simulink model "dp_controller"  (R2020a)
settings: Solver=FixedStepAuto  StartTime=0.0  StopTime=10.0  FixedStep=0.01  RelTol=1e-3
PreLoadFcn:
  | load("interfaces.mat");
undefined symbols (not defined in the file or in its folder): surge, sway, yaw
libraries: simulink x3
settings Model: Creator=thomas.evang  LastModifiedBy=thomas.evang
settings SFSimCC: CustomCodeUndefinedFunction=UseInterfaceOnly
settings RTWCC: Description=Generic Real-Time Target  RetainRTWFile=on

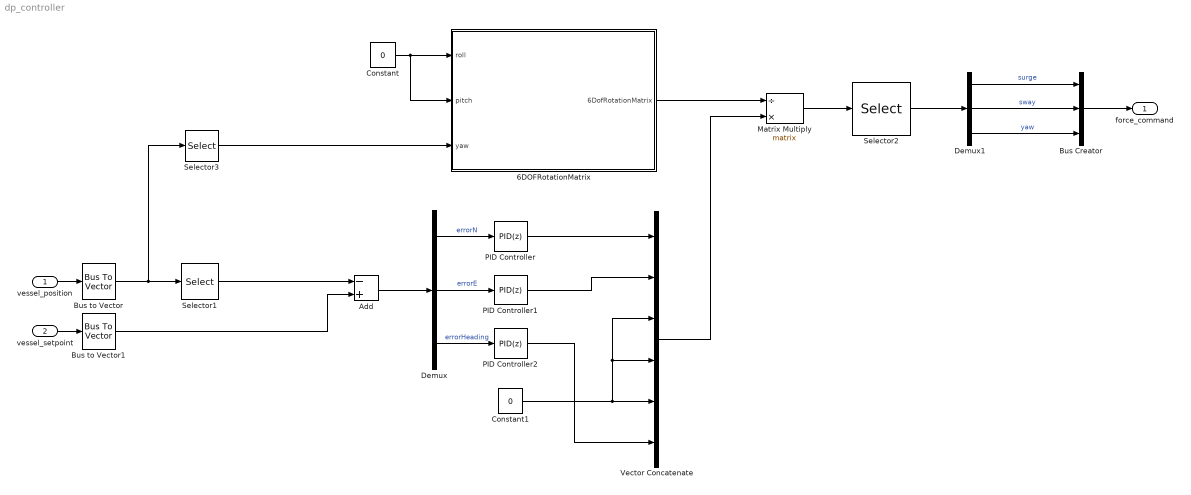
== system dp_controller ==
  vessel_position : Inport  OutDataTypeStr=Bus: position_6dof
  vessel_setpoint : Inport  Port=2  OutDataTypeStr=Bus: position_3dof
  6DOFRotationMatrix : Subsystem
  Add : Sum  Inputs=-+
  Bus Creator : BusCreator  Inputs=surge,sway,yaw  OutDataTypeStr=Bus: force_3dof
  Bus to Vector : BusToVector
  Bus to Vector1 : BusToVector
  Constant : Constant  Value=0
  Constant1 : Constant  Value=0
  Demux : Demux  Outputs=3
  Demux1 : Demux  Outputs=3
  Matrix Multiply : Product  Inputs=/*  Multiplication=Matrix(*)
  PID Controller : simulink/Continuous/PID Controller  Controller=PID  Form=Parallel  TimeDomain=Discrete-time  UseExternalTs=off  SampleTime=1e-1  IntegratorMethod=Forward Euler  FilterMethod=Forward Euler  ControllerParametersSource=internal  P=50000  I=100  D=5000000  UseFilter=off  N=0  TunerSelectOption=Transfer Function Based (PID Tuner App)  InitialConditionSource=internal  InitialConditionForIntegrator=0  InitialConditionForFilter=0  DifferentiatorICPrevScaledInput=0  ExternalReset=none  TrackingMode=off  Kt=1  LimitOutput=off  UpperSaturationLimit=inf  LowerSaturationLimit=-inf  LinearizeAsGain=on  AntiWindupMode=none  Kb=1  POutMin=[]  POutMax=[]  IOutMin=[]  IOutMax=[]  DOutMin=[]  DOutMax=[]  NOutMin=[]  NOutMax=[]  SumOutMin=[]  SumOutMax=[]  SaturationOutMin=[]  SaturationOutMax=[]  PParamMin=[]  PParamMax=[]  IParamMin=[]  IParamMax=[]  DParamMin=[]  DParamMax=[]  NParamMin=[]  NParamMax=[]  KbParamMin=[]  KbParamMax=[]  KtParamMin=[]  KtParamMax=[]  KbOutMin=[]  KbOutMax=[]  KtOutMin=[]  KtOutMax=[]  IntegratorOutMin=[]  IntegratorOutMax=[]  FilterOutMin=[]  FilterOutMax=[]  SumI1OutMin=[]  SumI1OutMax=[]  SumI2OutMin=[]  SumI2OutMax=[]  SumI3OutMin=[]  SumI3OutMax=[]  SumI4OutMin=[]  SumI4OutMax=[]  SumDOutMin=[]  SumDOutMax=[]  DifferentiatorOutMin=[]  DifferentiatorOutMax=[]  FilterDiffOutCoefMin=[]  FilterDiffOutCoefMax=[]  ReciprocalOutMin=[]  ReciprocalOutMax=[]  SumDenOutMin=[]  SumDenOutMax=[]  SumNumOutMin=[]  SumNumOutMax=[]  DivideOutMin=[]  DivideOutMax=[]  UdiffTsProdOutMin=[]  UdiffTsProdOutMax=[]  NTsProdOutMin=[]  NTsProdOutMax=[]  UintegralTsProdOutMin=[]  UintegralTsProdOutMax=[]  UngainTsProdOutMin=[]  UngainTsProdOutMax=[]  IntegratorContinuousStateAttributes=''  IntegratorStateMustResolveToSignalObject=off  IntegratorRTWStateStorageClass=Auto  FilterContinuousStateAttributes=''  FilterStateMustResolveToSignalObject=off  FilterRTWStateStorageClass=Auto  ParallelPVariant=InternalParameters  IdealPVariant=Disabled  IVariant=InternalParameters  DVariant=InternalParameters  IntegratorVariant=Discrete  SatVariant=Disabled  AWVariant=Passthrough  PCopyVariant=Disabled  TRVariant=Disabled  FdbkBlocksVariant=Forward  IdealPFdbkVariant=Disabled  SatFdbkVariant=Disabled  DerivativeFilterVariant=Differentiator  NVariant=Passthrough  NCopyVariant=Disabled_SignalSpec  FilterICVariant=InternalICsDifferentiator  IntegratorICVariant=InternalICs  ExternalResetVariant=Disabled  TRSumVariant=Passthrough  SumFdbkVariant=Disabled  SumVariant=Sum_PID  TsampFilterVariant=InternalTs  TsampNgainVariant=Passthrough  TsampIntegralVariant=Passthrough
  PID Controller1 : simulink/Continuous/PID Controller  Controller=PID  Form=Parallel  TimeDomain=Discrete-time  UseExternalTs=off  SampleTime=1e-1  IntegratorMethod=Forward Euler  FilterMethod=Forward Euler  ControllerParametersSource=internal  P=50000  I=100  D=5000000  UseFilter=off  N=0  TunerSelectOption=Transfer Function Based (PID Tuner App)  InitialConditionSource=internal  InitialConditionForIntegrator=0  InitialConditionForFilter=0  DifferentiatorICPrevScaledInput=0  ExternalReset=none  TrackingMode=off  Kt=1  LimitOutput=off  UpperSaturationLimit=inf  LowerSaturationLimit=-inf  LinearizeAsGain=on  AntiWindupMode=none  Kb=1  POutMin=[]  POutMax=[]  IOutMin=[]  IOutMax=[]  DOutMin=[]  DOutMax=[]  NOutMin=[]  NOutMax=[]  SumOutMin=[]  SumOutMax=[]  SaturationOutMin=[]  SaturationOutMax=[]  PParamMin=[]  PParamMax=[]  IParamMin=[]  IParamMax=[]  DParamMin=[]  DParamMax=[]  NParamMin=[]  NParamMax=[]  KbParamMin=[]  KbParamMax=[]  KtParamMin=[]  KtParamMax=[]  KbOutMin=[]  KbOutMax=[]  KtOutMin=[]  KtOutMax=[]  IntegratorOutMin=[]  IntegratorOutMax=[]  FilterOutMin=[]  FilterOutMax=[]  SumI1OutMin=[]  SumI1OutMax=[]  SumI2OutMin=[]  SumI2OutMax=[]  SumI3OutMin=[]  SumI3OutMax=[]  SumI4OutMin=[]  SumI4OutMax=[]  SumDOutMin=[]  SumDOutMax=[]  DifferentiatorOutMin=[]  DifferentiatorOutMax=[]  FilterDiffOutCoefMin=[]  FilterDiffOutCoefMax=[]  ReciprocalOutMin=[]  ReciprocalOutMax=[]  SumDenOutMin=[]  SumDenOutMax=[]  SumNumOutMin=[]  SumNumOutMax=[]  DivideOutMin=[]  DivideOutMax=[]  UdiffTsProdOutMin=[]  UdiffTsProdOutMax=[]  NTsProdOutMin=[]  NTsProdOutMax=[]  UintegralTsProdOutMin=[]  UintegralTsProdOutMax=[]  UngainTsProdOutMin=[]  UngainTsProdOutMax=[]  IntegratorContinuousStateAttributes=''  IntegratorStateMustResolveToSignalObject=off  IntegratorRTWStateStorageClass=Auto  FilterContinuousStateAttributes=''  FilterStateMustResolveToSignalObject=off  FilterRTWStateStorageClass=Auto  ParallelPVariant=InternalParameters  IdealPVariant=Disabled  IVariant=InternalParameters  DVariant=InternalParameters  IntegratorVariant=Discrete  SatVariant=Disabled  AWVariant=Passthrough  PCopyVariant=Disabled  TRVariant=Disabled  FdbkBlocksVariant=Forward  IdealPFdbkVariant=Disabled  SatFdbkVariant=Disabled  DerivativeFilterVariant=Differentiator  NVariant=Passthrough  NCopyVariant=Disabled_SignalSpec  FilterICVariant=InternalICsDifferentiator  IntegratorICVariant=InternalICs  ExternalResetVariant=Disabled  TRSumVariant=Passthrough  SumFdbkVariant=Disabled  SumVariant=Sum_PID  TsampFilterVariant=InternalTs  TsampNgainVariant=Passthrough  TsampIntegralVariant=Passthrough
  PID Controller2 : simulink/Continuous/PID Controller  Controller=PID  Form=Parallel  TimeDomain=Discrete-time  UseExternalTs=off  SampleTime=1e-1  IntegratorMethod=Forward Euler  FilterMethod=Forward Euler  ControllerParametersSource=internal  P=987355.105195486  I=621.647398453693  D=34853426.651765  UseFilter=off  N=100  TunerSelectOption=Transfer Function Based (PID Tuner App)  InitialConditionSource=internal  InitialConditionForIntegrator=0  InitialConditionForFilter=0  DifferentiatorICPrevScaledInput=0  ExternalReset=none  TrackingMode=off  Kt=1  LimitOutput=off  UpperSaturationLimit=inf  LowerSaturationLimit=-inf  LinearizeAsGain=on  AntiWindupMode=none  Kb=1  POutMin=[]  POutMax=[]  IOutMin=[]  IOutMax=[]  DOutMin=[]  DOutMax=[]  NOutMin=[]  NOutMax=[]  SumOutMin=[]  SumOutMax=[]  SaturationOutMin=[]  SaturationOutMax=[]  PParamMin=[]  PParamMax=[]  IParamMin=[]  IParamMax=[]  DParamMin=[]  DParamMax=[]  NParamMin=[]  NParamMax=[]  KbParamMin=[]  KbParamMax=[]  KtParamMin=[]  KtParamMax=[]  KbOutMin=[]  KbOutMax=[]  KtOutMin=[]  KtOutMax=[]  IntegratorOutMin=[]  IntegratorOutMax=[]  FilterOutMin=[]  FilterOutMax=[]  SumI1OutMin=[]  SumI1OutMax=[]  SumI2OutMin=[]  SumI2OutMax=[]  SumI3OutMin=[]  SumI3OutMax=[]  SumI4OutMin=[]  SumI4OutMax=[]  SumDOutMin=[]  SumDOutMax=[]  DifferentiatorOutMin=[]  DifferentiatorOutMax=[]  FilterDiffOutCoefMin=[]  FilterDiffOutCoefMax=[]  ReciprocalOutMin=[]  ReciprocalOutMax=[]  SumDenOutMin=[]  SumDenOutMax=[]  SumNumOutMin=[]  SumNumOutMax=[]  DivideOutMin=[]  DivideOutMax=[]  UdiffTsProdOutMin=[]  UdiffTsProdOutMax=[]  NTsProdOutMin=[]  NTsProdOutMax=[]  UintegralTsProdOutMin=[]  UintegralTsProdOutMax=[]  UngainTsProdOutMin=[]  UngainTsProdOutMax=[]  IntegratorContinuousStateAttributes=''  IntegratorStateMustResolveToSignalObject=off  IntegratorRTWStateStorageClass=Auto  FilterContinuousStateAttributes=''  FilterStateMustResolveToSignalObject=off  FilterRTWStateStorageClass=Auto  ParallelPVariant=InternalParameters  IdealPVariant=Disabled  IVariant=InternalParameters  DVariant=InternalParameters  IntegratorVariant=Discrete  SatVariant=Disabled  AWVariant=Passthrough  PCopyVariant=Disabled  TRVariant=Disabled  FdbkBlocksVariant=Forward  IdealPFdbkVariant=Disabled  SatFdbkVariant=Disabled  DerivativeFilterVariant=Differentiator  NVariant=Passthrough  NCopyVariant=Disabled_SignalSpec  FilterICVariant=InternalICsDifferentiator  IntegratorICVariant=InternalICs  ExternalResetVariant=Disabled  TRSumVariant=Passthrough  SumFdbkVariant=Disabled  SumVariant=Sum_PID  TsampFilterVariant=InternalTs  TsampNgainVariant=Passthrough  TsampIntegralVariant=Passthrough
  Selector1 : Selector  InputPortWidth=6  IndexOptions=Index vector (dialog)  Indices=[1 2 6]  OutputSizes=1
  Selector2 : Selector  InputPortWidth=6  IndexOptions=Index vector (dialog)  Indices=[1 2 6]  OutputSizes=1
  Selector3 : Selector  InputPortWidth=6  IndexOptions=Index vector (dialog)  Indices=6  OutputSizes=1
  Vector Concatenate : Concatenate  NumInputs=6
  force_command : Outport  OutDataTypeStr=Bus: force_3dof  VectorParamsAs1DForOutWhenUnconnected=off
  wires:
  Selector1/1 -> Add/1
  PID Controller2/1 -> Vector Concatenate/6
  Matrix Multiply/1 -> Selector2/1
  Selector3/1 -> 6DOFRotationMatrix/3(yaw)
  Demux/1 -> PID Controller/1  "errorN"
  Demux/3 -> PID Controller2/1  "errorHeading"
  PID Controller/1 -> Vector Concatenate/1
  Add/1 -> Demux/1
  Constant/1 -> 6DOFRotationMatrix/1(roll), 6DOFRotationMatrix/2(pitch)
  vessel_setpoint/1 -> Bus to Vector1/1
  Constant1/1 -> Vector Concatenate/5, Vector Concatenate/3, Vector Concatenate/4
  PID Controller1/1 -> Vector Concatenate/2
  vessel_position/1 -> Bus to Vector/1
  Demux/2 -> PID Controller1/1  "errorE"
  Vector Concatenate/1 -> Matrix Multiply/2
  6DOFRotationMatrix/1(6DofRotationMatrix) -> Matrix Multiply/1
  Selector2/1 -> Demux1/1
  Bus Creator/1 -> force_command/1
  Demux1/1 -> Bus Creator/1  "surge"
  Demux1/2 -> Bus Creator/2  "sway"
  Demux1/3 -> Bus Creator/3  "yaw"
  Bus to Vector/1 -> Selector3/1, Selector1/1
  Bus to Vector1/1 -> Add/2

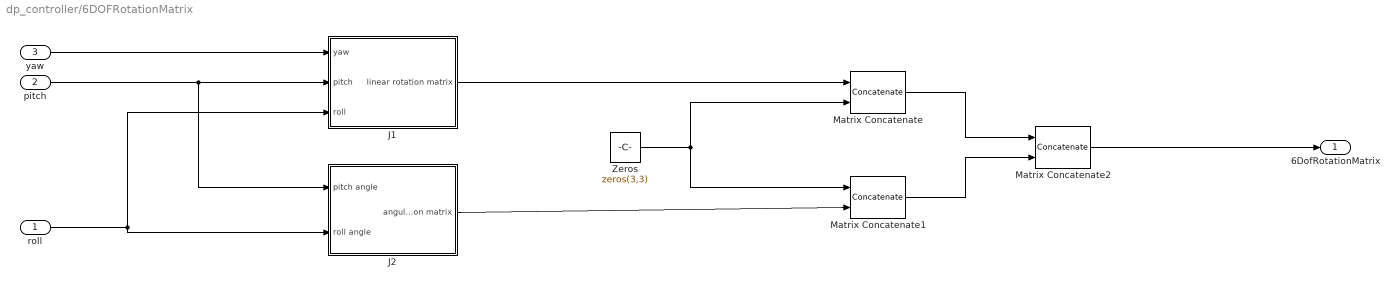
== system dp_controller/6DOFRotationMatrix ==
  roll : Inport
  pitch : Inport  Port=2
  yaw : Inport  Port=3
  J1 : Subsystem
  J2 : Subsystem
  Matrix Concatenate : Concatenate  Mode=Multidimensional array
  Matrix Concatenate1 : Concatenate  Mode=Multidimensional array
  Matrix Concatenate2 : Concatenate  Mode=Multidimensional array  ConcatenateDimension=2
  Zeros : Constant  Value=zeros(3,3)
  6DofRotationMatrix : Outport  VectorParamsAs1DForOutWhenUnconnected=off
  wires:
  J1/1(linear rotation matrix) -> Matrix Concatenate/1
  yaw/1 -> J1/1(yaw)
  J2/1(angular rotation matrix) -> Matrix Concatenate1/2
  Matrix Concatenate2/1 -> 6DofRotationMatrix/1
  Matrix Concatenate/1 -> Matrix Concatenate2/1
  Matrix Concatenate1/1 -> Matrix Concatenate2/2
  Zeros/1 -> Matrix Concatenate1/1, Matrix Concatenate/2
  roll/1 -> J2/2(roll angle), J1/3(roll)
  pitch/1 -> J1/2(pitch), J2/1(pitch angle)

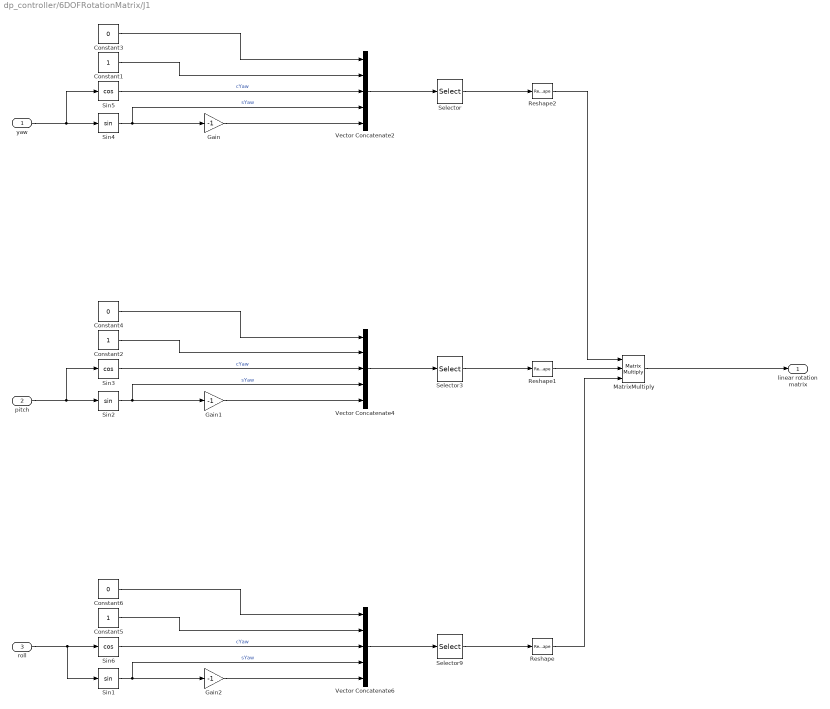
== system dp_controller/6DOFRotationMatrix/J1 ==
  yaw : Inport
  pitch : Inport  Port=2
  roll : Inport  Port=3
  Constant1 : Constant
  Constant2 : Constant
  Constant3 : Constant  Value=0
  Constant4 : Constant  Value=0
  Constant5 : Constant
  Constant6 : Constant  Value=0
  Gain : Gain  Gain=-1
  Gain1 : Gain  Gain=-1
  Gain2 : Gain  Gain=-1
  MatrixMultiply : Product  Inputs=3  Multiplication=Matrix(*)
  Reshape : Reshape  OutputDimensionality=Customize  OutputDimensions=[3,3]
  Reshape1 : Reshape  OutputDimensionality=Customize  OutputDimensions=[3,3]
  Reshape2 : Reshape  OutputDimensionality=Customize  OutputDimensions=[3,3]
  Selector : Selector  InputPortWidth=5  IndexOptions=Index vector (dialog)  Indices=[3 4 1 5 3 1 1 1 2]  OutputSizes=1
  Selector3 : Selector  InputPortWidth=5  IndexOptions=Index vector (dialog)  Indices=[3 1 5 1 2 1 4 1 3]  OutputSizes=1
  Selector9 : Selector  InputPortWidth=5  IndexOptions=Index vector (dialog)  Indices=[2 1 1 1 3 4 1 5 3]  OutputSizes=1
  Sin1 : Trigonometry
  Sin2 : Trigonometry
  Sin3 : Trigonometry  Operator=cos
  Sin4 : Trigonometry
  Sin5 : Trigonometry  Operator=cos
  Sin6 : Trigonometry  Operator=cos
  Vector Concatenate2 : Concatenate  NumInputs=5
  Vector Concatenate4 : Concatenate  NumInputs=5
  Vector Concatenate6 : Concatenate  NumInputs=5
  linear rotation matrix : Outport  VectorParamsAs1DForOutWhenUnconnected=off
  wires:
  Sin5/1 -> Vector Concatenate2/3  "cYaw"
  Constant3/1 -> Vector Concatenate2/1
  Constant2/1 -> Vector Concatenate4/2
  Constant4/1 -> Vector Concatenate4/1
  Gain1/1 -> Vector Concatenate4/5
  roll/1 -> Sin6/1, Sin1/1
  Constant1/1 -> Vector Concatenate2/2
  Vector Concatenate4/1 -> Selector3/1
  Vector Concatenate2/1 -> Selector/1
  Reshape2/1 -> MatrixMultiply/1
  Gain/1 -> Vector Concatenate2/5
  Selector9/1 -> Reshape/1
  Vector Concatenate6/1 -> Selector9/1
  Gain2/1 -> Vector Concatenate6/5
  Reshape1/1 -> MatrixMultiply/2
  Selector3/1 -> Reshape1/1
  Sin4/1 -> Gain/1, Vector Concatenate2/4  "sYaw"
  Sin6/1 -> Vector Concatenate6/3  "cYaw"
  Sin2/1 -> Vector Concatenate4/4, Gain1/1  "sYaw"
  Reshape/1 -> MatrixMultiply/3
  yaw/1 -> Sin4/1, Sin5/1
  Selector/1 -> Reshape2/1
  Sin1/1 -> Gain2/1, Vector Concatenate6/4  "sYaw"
  MatrixMultiply/1 -> linear rotation matrix/1
  Constant5/1 -> Vector Concatenate6/2
  Sin3/1 -> Vector Concatenate4/3  "cYaw"
  Constant6/1 -> Vector Concatenate6/1
  pitch/1 -> Sin2/1, Sin3/1

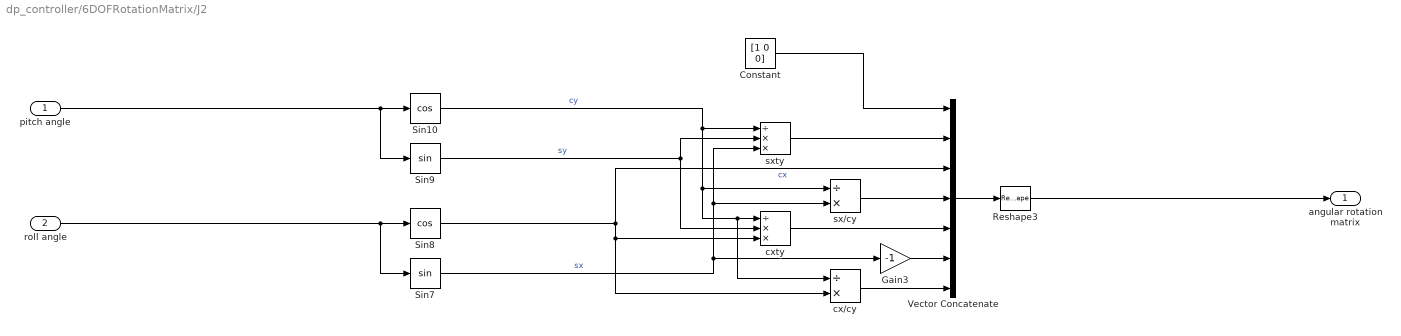
== system dp_controller/6DOFRotationMatrix/J2 ==
  pitch angle : Inport
  roll angle : Inport  Port=2
  Constant : Constant  Value=[1 0 0]
  Gain3 : Gain  Gain=-1
  Reshape3 : Reshape  OutputDimensionality=Customize  OutputDimensions=[3,3]
  Sin10 : Trigonometry  Operator=cos
  Sin7 : Trigonometry
  Sin8 : Trigonometry  Operator=cos
  Sin9 : Trigonometry
  Vector Concatenate : Concatenate  NumInputs=7
  cx/cy : Product  Inputs=/*
  cxty : Product  Inputs=/**
  sx/cy : Product  Inputs=/*
  sxty : Product  Inputs=/**
  angular rotation matrix : Outport  VectorParamsAs1DForOutWhenUnconnected=off
  wires:
  Reshape3/1 -> angular rotation matrix/1
  Gain3/1 -> Vector Concatenate/6
  Constant/1 -> Vector Concatenate/1
  Sin10/1 -> sxty/1, cxty/1, cx/cy/1, sx/cy/1  "cy"
  Vector Concatenate/1 -> Reshape3/1
  cx/cy/1 -> Vector Concatenate/7
  sx/cy/1 -> Vector Concatenate/4
  Sin8/1 -> Vector Concatenate/3, cxty/3, cx/cy/2  "cx"
  cxty/1 -> Vector Concatenate/5
  roll angle/1 -> Sin8/1, Sin7/1
  Sin9/1 -> sxty/2, cxty/2  "sy"
  sxty/1 -> Vector Concatenate/2
  pitch angle/1 -> Sin10/1, Sin9/1
  Sin7/1 -> Gain3/1, sx/cy/2, sxty/3  "sx"
